simulink model "trajectory_tracking_simulation_on_kinematic_model_R2019b"  (R2019b)
settings: Solver=VariableStepAuto  StartTime=0.0  StopTime=20  RelTol=1e-3
InitFcn:
  | parameters_for_trajectory_tracking_simulation
StopFcn:
  | plot_trajectory_at_simulation_stop(out,true,0.5*half_wheel_base_for_model,false)
model workspace (MAT data in the model file):
  Current_Seg = Simulink.Signal
  Current_Seg.DataType = 'uint8'
  Current_Seg.Dimensions = -1
  Current_Seg.DimensionsMode = 'auto'
  Current_Seg.Complexity = 'auto'
  Current_Seg.SampleTime = -1
  Current_Seg.SamplingMode = 'auto'
  Current_Seg.InitialValue = '1'
  Current_Segment = Simulink.Signal
  Current_Segment.DataType = 'uint8'
  Current_Segment.Dimensions = -1
  Current_Segment.DimensionsMode = 'Fixed'
  Current_Segment.Complexity = 'real'
  Current_Segment.SampleTime = -1
  Current_Segment.SamplingMode = 'auto'
  Current_Segment.InitialValue = '0'
  Locked_Pos = Simulink.Signal
  Locked_Pos.DataType = 'uint8'
  Locked_Pos.Dimensions = -1
  Locked_Pos.DimensionsMode = 'auto'
  Locked_Pos.Complexity = 'auto'
  Locked_Pos.SampleTime = -1
  Locked_Pos.SamplingMode = 'auto'
  Locked_Pos.InitialValue = '0'
values from neighbouring files (symbols this model uses):
  half_wheel_base_for_controller = 0.125    [parameters_for_trajectory_tracking_simulation.m]
  half_wheel_base_for_model = 0.125    [parameters_for_trajectory_tracking_simulation.m]
  odometry_phi_initial = phi_initial    (= 0)    [parameters_for_trajectory_tracking_simulation.m]
  odometry_pose_covariance_initial = zeros(3,3)    [parameters_for_trajectory_tracking_simulation.m]
  odometry_theta_l_variance_scaling = (0.05)^2    (= 0.0025)    [parameters_for_trajectory_tracking_simulation.m]
  odometry_theta_r_variance_scaling = (0.05)^2    (= 0.0025)    [parameters_for_trajectory_tracking_simulation.m]
  odometry_x_p_initial = x_p_initial    (= 0.5)    [parameters_for_trajectory_tracking_simulation.m]
  odometry_y_p_initial = y_p_initial    (= 3)    [parameters_for_trajectory_tracking_simulation.m]
  phi_initial = 0 * (pi/180)    (= 0)    [development_of_path_planning.m]    (also in parameters_for_trajectory_tracking_simulation.m; path_planning_and_trajectory_generation.m = pose_initial(3))
  theta_l_initial = 0    [parameters_for_trajectory_tracking_simulation.m]
  theta_r_initial = 0    [parameters_for_trajectory_tracking_simulation.m]
  trajectory_description = [0.5, 3, 1, 3.5, pi/4 ... (first row only)    [path_planning_and_trajectory_generation.m]
  wheel_radius_left_for_controller = 0.050    (= 0.05)    [parameters_for_trajectory_tracking_simulation.m]
  wheel_radius_left_for_model = 0.050    (= 0.05)    [parameters_for_trajectory_tracking_simulation.m]
  wheel_radius_right_for_controller = 0.050    (= 0.05)    [parameters_for_trajectory_tracking_simulation.m]
  wheel_radius_right_for_model = 0.050    (= 0.05)    [parameters_for_trajectory_tracking_simulation.m]
  x_p_initial = 0.5    [development_of_path_planning.m]    (also in parameters_for_trajectory_tracking_simulation.m; path_planning_and_trajectory_generation.m = pose_initial(1))
  y_p_initial = 3.0    (= 3)    [development_of_path_planning.m]    (also in parameters_for_trajectory_tracking_simulation.m; path_planning_and_trajectory_generation.m = pose_initial(2))
settings Model: Creator=pbeuchat  LastModifiedBy=nicpa

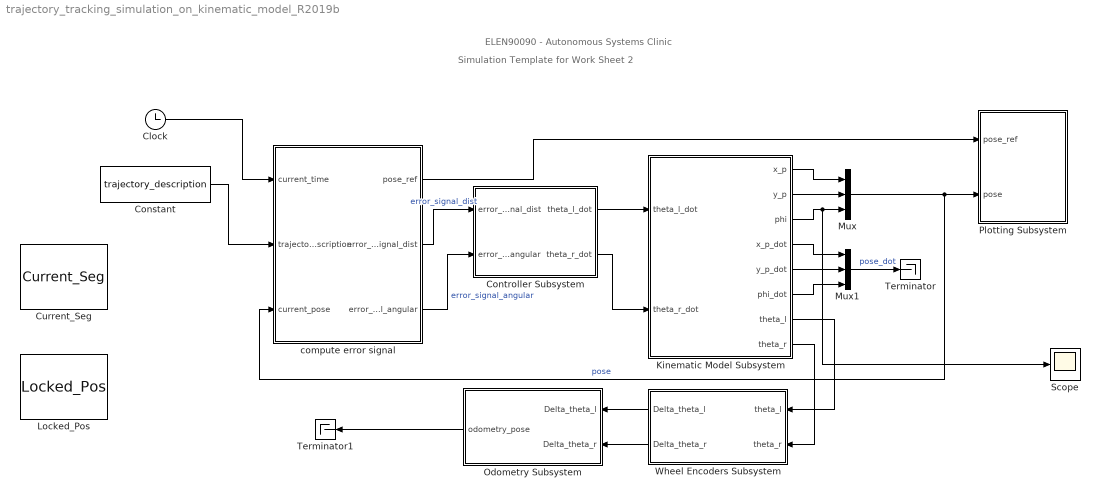
== system trajectory_tracking_simulation_on_kinematic_model_R2019b ==
  note: ELEN90090 - Autonomous Systems Clinic
  note: Simulation Template for Work Sheet 2
  Clock : Clock
  Constant : Constant  Value=trajectory_description
  Controller Subsystem : Subsystem
  Current_Seg : DataStoreMemory  DataStoreName=Current_Seg  ReadBeforeWriteMsg=warning  WriteAfterWriteMsg=warning  WriteAfterReadMsg=warning  InitialValue=1  ShowAdditionalParam=off  OutDataTypeStr=uint8  StateMustResolveToSignalObject=on
  Kinematic Model Subsystem : Subsystem
  Locked_Pos : DataStoreMemory  DataStoreName=Locked_Pos  ReadBeforeWriteMsg=warning  WriteAfterWriteMsg=warning  WriteAfterReadMsg=warning  ShowAdditionalParam=off  OutDataTypeStr=uint8  StateMustResolveToSignalObject=on
  Mux : Mux  Inputs=3
  Mux1 : Mux  Inputs=3
  Odometry Subsystem : Subsystem
  Plotting Subsystem : Subsystem
  Scope : Scope
  Terminator : Terminator
  Terminator1 : Terminator
  Wheel Encoders Subsystem : Subsystem
  compute error signal : MATLAB Function  TreatAsAtomicUnit=on
  wires:
  Kinematic Model Subsystem/1(x_p) -> Mux/1
  Kinematic Model Subsystem/2(y_p) -> Mux/2
  Mux/1 -> compute error signal/3(current_pose), Plotting Subsystem/2(pose)  "pose"
  Kinematic Model Subsystem/4(x_p_dot) -> Mux1/1
  Kinematic Model Subsystem/5(y_p_dot) -> Mux1/2
  Kinematic Model Subsystem/6(phi_dot) -> Mux1/3
  Mux1/1 -> Terminator/1  "pose_dot"
  compute error signal/2(error_signal_dist) -> Controller Subsystem/1("error_signal_dist ")  "error_signal_dist"
  Controller Subsystem/1(theta_l_dot) -> Kinematic Model Subsystem/1(theta_l_dot)
  Controller Subsystem/2(theta_r_dot) -> Kinematic Model Subsystem/2(theta_r_dot)
  compute error signal/1(pose_ref) -> Plotting Subsystem/1(pose_ref)
  Clock/1 -> compute error signal/1(current_time)
  Constant/1 -> compute error signal/2(trajectory_description)
  Kinematic Model Subsystem/7(theta_l) -> Wheel Encoders Subsystem/1(theta_l)
  Kinematic Model Subsystem/8(theta_r) -> Wheel Encoders Subsystem/2(theta_r)
  Wheel Encoders Subsystem/1(Delta_theta_l) -> Odometry Subsystem/1(Delta_theta_l)
  Wheel Encoders Subsystem/2(Delta_theta_r) -> Odometry Subsystem/2(Delta_theta_r)
  Odometry Subsystem/1(odometry_pose) -> Terminator1/1
  compute error signal/3(error_signal_angular) -> Controller Subsystem/2("error_signal_angular ")  "error_signal_angular"
  Kinematic Model Subsystem/3(phi) -> Scope/1, Mux/3

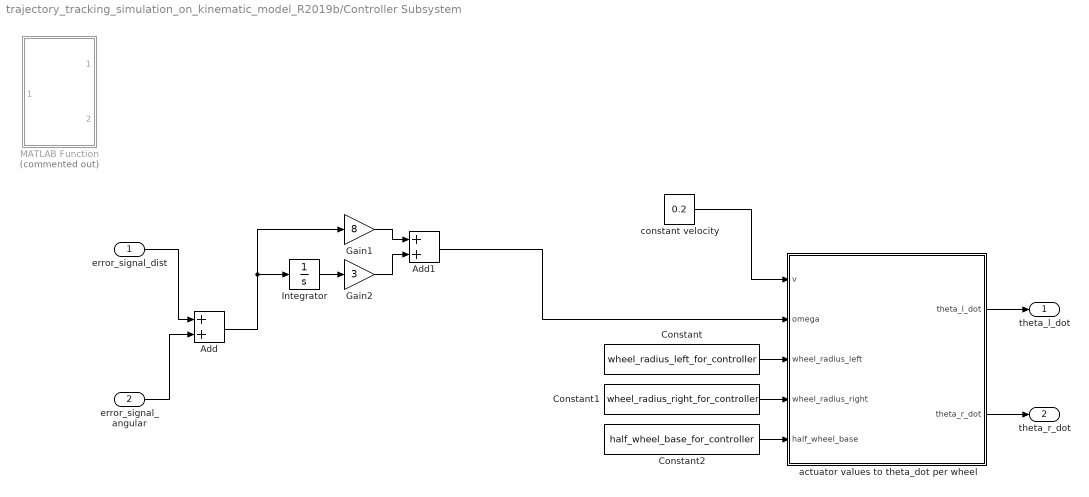
== system trajectory_tracking_simulation_on_kinematic_model_R2019b/Controller Subsystem ==
  "error_signal_dist " : Inport
  "error_signal_angular " : Inport  Port=2
  Add : Sum
  Add1 : Sum
  Constant : Constant  Value=wheel_radius_left_for_controller
  Constant1 : Constant  Value=wheel_radius_right_for_controller
  Constant2 : Constant  Value=half_wheel_base_for_controller
  Gain1 : Gain  Gain=8
  Gain2 : Gain  Gain=3
  Integrator : Integrator
  MATLAB Function : MATLAB Function  Commented=on  TreatAsAtomicUnit=on
  actuator values to theta_dot per wheel : MATLAB Function  TreatAsAtomicUnit=on
  "constant velocity " : Constant  Value=0.2  OutDataTypeStr=Inherit: Inherit via back propagation
  theta_l_dot : Outport
  theta_r_dot : Outport  Port=2
  wires:
  Constant/1 -> actuator values to theta_dot per wheel/3(wheel_radius_left)
  actuator values to theta_dot per wheel/2(theta_r_dot) -> theta_r_dot/1
  actuator values to theta_dot per wheel/1(theta_l_dot) -> theta_l_dot/1
  Constant2/1 -> actuator values to theta_dot per wheel/5(half_wheel_base)
  Constant1/1 -> actuator values to theta_dot per wheel/4(wheel_radius_right)
  "constant velocity "/1 -> actuator values to theta_dot per wheel/1(v)
  Add1/1 -> actuator values to theta_dot per wheel/2(omega)
  "error_signal_angular "/1 -> Add/2
  Integrator/1 -> Gain2/1
  Gain1/1 -> Add1/1
  Gain2/1 -> Add1/2
  "error_signal_dist "/1 -> Add/1
  Add/1 -> Gain1/1, Integrator/1

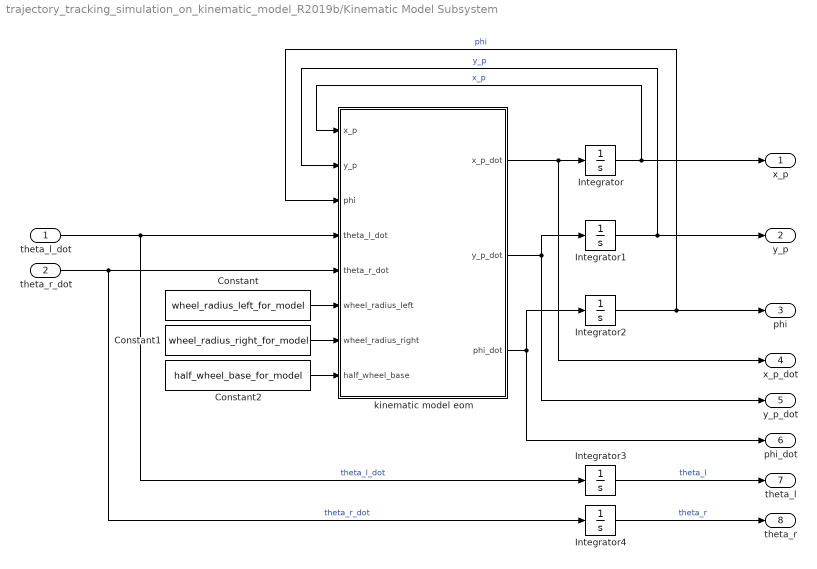
== system trajectory_tracking_simulation_on_kinematic_model_R2019b/Kinematic Model Subsystem ==
  theta_l_dot : Inport
  theta_r_dot : Inport  Port=2
  Constant : Constant  Value=wheel_radius_left_for_model
  Constant1 : Constant  Value=wheel_radius_right_for_model
  Constant2 : Constant  Value=half_wheel_base_for_model
  Integrator : Integrator  InitialCondition=x_p_initial
  Integrator1 : Integrator  InitialCondition=y_p_initial
  Integrator2 : Integrator  InitialCondition=phi_initial
  Integrator3 : Integrator  InitialCondition=theta_l_initial
  Integrator4 : Integrator  InitialCondition=theta_r_initial
  kinematic model eom : MATLAB Function  TreatAsAtomicUnit=on
  x_p : Outport
  y_p : Outport  Port=2
  phi : Outport  Port=3
  x_p_dot : Outport  Port=4
  y_p_dot : Outport  Port=5
  phi_dot : Outport  Port=6
  theta_l : Outport  Port=7
  theta_r : Outport  Port=8
  wires:
  theta_l_dot/1 -> kinematic model eom/4(theta_l_dot), Integrator3/1  "theta_l_dot"
  Integrator/1 -> kinematic model eom/1(x_p), x_p/1  "x_p"
  Constant1/1 -> kinematic model eom/7(wheel_radius_right)
  theta_r_dot/1 -> Integrator4/1, kinematic model eom/5(theta_r_dot)  "theta_r_dot"
  Constant/1 -> kinematic model eom/6(wheel_radius_left)
  kinematic model eom/1(x_p_dot) -> x_p_dot/1, Integrator/1
  kinematic model eom/2(y_p_dot) -> y_p_dot/1, Integrator1/1
  kinematic model eom/3(phi_dot) -> phi_dot/1, Integrator2/1
  Integrator1/1 -> y_p/1, kinematic model eom/2(y_p)  "y_p"
  Integrator2/1 -> phi/1, kinematic model eom/3(phi)  "phi"
  Constant2/1 -> kinematic model eom/8(half_wheel_base)
  Integrator4/1 -> theta_r/1  "theta_r"
  Integrator3/1 -> theta_l/1  "theta_l"

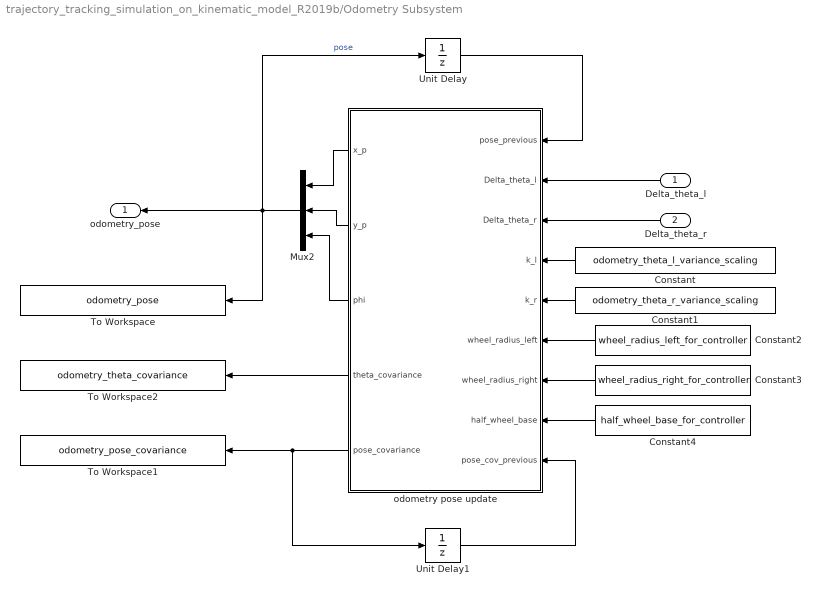
== system trajectory_tracking_simulation_on_kinematic_model_R2019b/Odometry Subsystem ==
  Delta_theta_l : Inport
  Delta_theta_r : Inport  Port=2
  Constant : Constant  Value=odometry_theta_l_variance_scaling
  Constant1 : Constant  Value=odometry_theta_r_variance_scaling
  Constant2 : Constant  Value=wheel_radius_left_for_controller
  Constant3 : Constant  Value=wheel_radius_right_for_controller
  Constant4 : Constant  Value=half_wheel_base_for_controller
  Mux2 : Mux  Inputs=3
  To Workspace : ToWorkspace  VariableName=odometry_pose  SaveFormat=Timeseries  SampleTime=-1
  To Workspace1 : ToWorkspace  VariableName=odometry_pose_covariance  SaveFormat=Timeseries  SampleTime=-1
  To Workspace2 : ToWorkspace  VariableName=odometry_theta_covariance  SaveFormat=Timeseries  SampleTime=-1
  Unit Delay : UnitDelay  InitialCondition=[odometry_x_p_initial;odometry_y_p_initial;odometry_phi_initial]  SampleTime=-1  HasFrameUpgradeWarning=on
  Unit Delay1 : UnitDelay  InitialCondition=odometry_pose_covariance_initial  SampleTime=-1  HasFrameUpgradeWarning=on
  odometry pose update : MATLAB Function  TreatAsAtomicUnit=on
  odometry_pose : Outport
  wires:
  Delta_theta_l/1 -> odometry pose update/2(Delta_theta_l)
  Delta_theta_r/1 -> odometry pose update/3(Delta_theta_r)
  odometry pose update/2(y_p) -> Mux2/2
  odometry pose update/1(x_p) -> Mux2/1
  Mux2/1 -> Unit Delay/1, odometry_pose/1, To Workspace/1  "pose"
  odometry pose update/3(phi) -> Mux2/3
  Unit Delay/1 -> odometry pose update/1(pose_previous)
  odometry pose update/5(pose_covariance) -> Unit Delay1/1, To Workspace1/1
  odometry pose update/4(theta_covariance) -> To Workspace2/1
  Constant/1 -> odometry pose update/4(k_l)
  Constant1/1 -> odometry pose update/5(k_r)
  Constant2/1 -> odometry pose update/6(wheel_radius_left)
  Constant3/1 -> odometry pose update/7(wheel_radius_right)
  Constant4/1 -> odometry pose update/8(half_wheel_base)
  Unit Delay1/1 -> odometry pose update/9(pose_cov_previous)

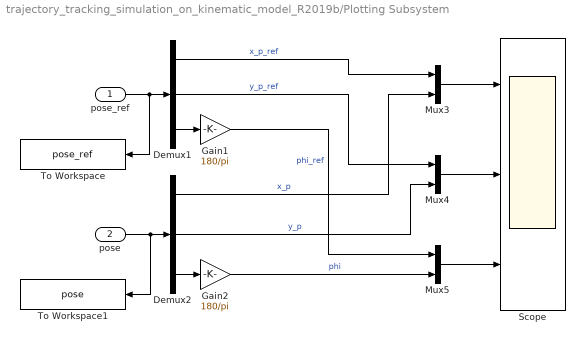
== system trajectory_tracking_simulation_on_kinematic_model_R2019b/Plotting Subsystem ==
  pose_ref : Inport
  pose : Inport  Port=2
  Demux1 : Demux  Outputs=3
  Demux2 : Demux  Outputs=3
  Gain1 : Gain  Gain=180/pi
  Gain2 : Gain  Gain=180/pi
  Mux3 : Mux  Inputs=2
  Mux4 : Mux  Inputs=2
  Mux5 : Mux  Inputs=2
  Scope : Scope  NumInputPorts=3
  To Workspace : ToWorkspace  VariableName=pose_ref  SaveFormat=Timeseries  SampleTime=-1
  To Workspace1 : ToWorkspace  VariableName=pose  SaveFormat=Timeseries  SampleTime=-1
  wires:
  Demux2/3 -> Gain2/1
  Mux3/1 -> Scope/1
  Gain2/1 -> Mux5/2  "phi"
  Demux1/3 -> Gain1/1
  Gain1/1 -> Mux5/1  "phi_ref"
  Mux5/1 -> Scope/3
  Demux2/2 -> Mux4/2  "y_p"
  pose/1 -> To Workspace1/1, Demux2/1
  Mux4/1 -> Scope/2
  Demux1/2 -> Mux4/1  "y_p_ref"
  Demux2/1 -> Mux3/2  "x_p"
  Demux1/1 -> Mux3/1  "x_p_ref"
  pose_ref/1 -> To Workspace/1, Demux1/1

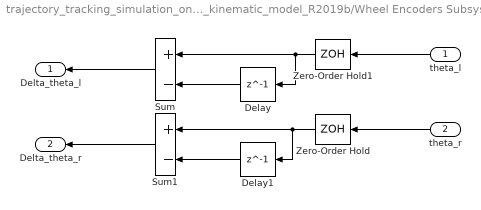
== system trajectory_tracking_simulation_on_kinematic_model_R2019b/Wheel Encoders Subsystem ==
  theta_l : Inport
  theta_r : Inport  Port=2
  Delay : Delay  DelayLength=1
  Delay1 : Delay  DelayLength=1
  Sum : Sum  Inputs=+-
  Sum1 : Sum  Inputs=+-
  Zero-Order Hold : ZeroOrderHold  SampleTime=0.01
  Zero-Order Hold1 : ZeroOrderHold  SampleTime=0.01
  Delta_theta_l : Outport
  Delta_theta_r : Outport  Port=2
  wires:
  theta_l/1 -> Zero-Order Hold1/1
  Sum1/1 -> Delta_theta_r/1
  theta_r/1 -> Zero-Order Hold/1
  Delay1/1 -> Sum1/2
  Zero-Order Hold/1 -> Sum1/1, Delay1/1
  Delay/1 -> Sum/2
  Sum/1 -> Delta_theta_l/1
  Zero-Order Hold1/1 -> Delay/1, Sum/1

== matlab function trajectory_tracking_simulation_on_kinematic_model_R2019b/Controller Subsystem/actuator values to theta_dot per wheel ==
  data: v input; theta_l_dot output; omega input; wheel_radius_left input; wheel_radius_right input; theta_r_dot output; half_wheel_base input
function [theta_l_dot , theta_r_dot] = ...
    actuators_to_theta_dot(...
        v ,...
        omega ,...
        wheel_radius_left ,...
        wheel_radius_right ,...
        half_wheel_base ...
    )
%  ---------------------------------------------------------------------  %
%% DESCRIPTION: THIS FUNCTION SHOULD CONVERT THE "v" AND "omega" ACTUATORS
%% TO DESIRED ANGULAR VELOCITY OF EACH WHEEL
%
%  INPUT ARGUMENTS:
%  v                    Forward velocity of the robot, in meters/second
%  omega                Angular velocity of the robot, in radians/second
%  wheel_radius_left    Radius of the left-hand wheel, in meters
%  wheel_radius_right   Radius of the right-hand wheel, in meters
%  half_wheel_base      Half the distance between the wheels, in meters
%
%  RETURN VARIABLES:
%  theta_l_dot    Angular velocity of the left-hand wheel, in radians/second
%  theta_r_dot    Angular velocity of the right-hand wheel, in radians/second
%
%  ---------------------------------------------------------------------  %

%% REPLACE THE CODE BELOW WITH THE CONVERSION
%simplified actuation

theta_l_dot = (v / wheel_radius_left) - (half_wheel_base * omega / wheel_radius_left);
%theta_l_dot = (v / wheel_radius_left);

theta_r_dot = (v / wheel_radius_right) + (half_wheel_base * omega / wheel_radius_right);

% %symbolic variables for equations solving 
% syms theta_l_dot_sym theta_r_dot_sym
% 
% %set up simultaneous equations
% eqn1 = (wheel_radius_left * theta_l_dot_sym / 2) + (wheel_radius_right * theta_r_dot_sym / 2) == v;
% eqn2 = (wheel_radius_right * theta_r_dot_sym / (2 * half_wheel_base)) - (wheel_radius_left * theta_l_dot_sym / (2 * half_wheel_base)) == omega;
% 
% %solve simultaneous equations 
% sol = solve([eqn1 eqn2], [theta_l_dot_sym theta_r_dot_sym]);
% 
% theta_l_dot = sol.theta_l_dot_sym;
% theta_r_dot = sol.theta_r_dot_sym;

== matlab function trajectory_tracking_simulation_on_kinematic_model_R2019b/Kinematic Model Subsystem/kinematic model eom ==
  data: x_p input; x_p_dot output; y_p input; phi input; theta_l_dot input; theta_r_dot input; y_p_dot output; phi_dot output; wheel_radius_left input; wheel_radius_right input; half_wheel_base input
function [x_p_dot,y_p_dot,phi_dot] = ...
    kinematic_model_eom(...
        x_p ,...
        y_p ,...
        phi ,...
        theta_l_dot ,...
        theta_r_dot ,...
        wheel_radius_left ,...
        wheel_radius_right ,...
        half_wheel_base ...
    )
%  ---------------------------------------------------------------------  %
%% DESCRIPTION: THIS FUNCTION SHOULD IMPLEMENT THE EQUATIONS OF MOTION
%% FOR THE KINEMATIC MODEL
%
%  INPUT ARGUMENTS:
%  x_p                  Intertial frame x-coordinate of the robot
%  y_p                  Intertial frame y-coordinate of the robot
%  phi                  Heading angle of the robot, in radians
%  theta_l_dot          Angular velocity of the left-hand wheel, in radians/second
%  theta_r_dot          Angular velocity of the right-hand wheel, in radians/second
%  wheel_radius_left    Radius of the left-hand wheel, in meters
%  wheel_radius_right   Radius of the right-hand wheel, in meters
%  half_wheel_base      Half the distance between the wheels, in meters
%
%  RETURN VARIABLES:
%  x_p_dot    Intertial frame x-coordinate velocity of the robot
%  y_p_dot    Intertial frame y-coordinate velocity of the robot
%  phi_dot    Heading anglular velocity of the robot
%
%  ---------------------------------------------------------------------  %

%% REAPLCE THE CODE BELOW WITH THE KINEMATIC MODEL
%transform from body frame to inertial frame
R_body_inertial = [cos(phi) -sin(phi) 0; sin(phi) cos(phi) 0; 0 0 1];

%note: assuming wheel_radius_left and wheel_radius right are the same. ALSO
%IF THEY ARENT THE SAME THIS MAY NOT BE THE CORRECT WAY TO PUT IT IN
wheel_params_matrix = [wheel_radius_left/2 wheel_radius_right/2; 0 0; 
    -wheel_radius_left/(2*half_wheel_base) wheel_radius_right/(2*half_wheel_base)];

wheel_velocities = [theta_l_dot; theta_r_dot];

velocities = R_body_inertial * wheel_params_matrix * wheel_velocities;


x_p_dot = velocities(1);
y_p_dot = velocities(2);
phi_dot = velocities(3);

== matlab function trajectory_tracking_simulation_on_kinematic_model_R2019b/compute error signal ==
  settings: updateMethod=DISCRETE
  data: pose_ref output; current_time input; trajectory_description input; error_signal_dist output; current_pose input; Current_Seg data_store_memory; Locked_Pos data_store_memory; error_signal_angular output
function [pose_ref , error_signal_dist, error_signal_angular] = ...
    compute_error_signal(...
        current_time ,...
        trajectory_description, ...
        current_pose)...
%  ---------------------------------------------------------------------  %
%% DESCRIPTION: THIS FUNCTION SHOULD GENERATE AN ERROR SIGNAL FOR X, Y AND THE HEADING
%
%  INPUT ARGUMENTS:
%  current_time    The current simulation time, in seconds
%
%  trajectory_description
%                  This is a matrix that specifies the interconnection of
%                  straight line segments that define the trajectory to
%                  follow as a function of time. Each row corresponds to a
%                  line segment, describing the start and end point of 
%                  the segment and the target heading i.e. each row is:
%                  [start_x start_y end_x end_y heading]
%
%  current_pose    A column vector of length 3 with the current pose of the
%                  robot, i.e.:
%                  current_pose(1) = x_p measurement, in meters
%                  current_pose(2) = y_p measurement, in meters
%                  current_pose(3) = heading angle measurement, in radians
%
% RETURN VARIABLE:
% pose_ref        A column vecotr of length 3 with the current reference
%                 along the trajectory, i.e.:
%                 pose_ref(1) = reference for x_p, in meters
%                 pose_ref(2) = reference for y_p, in meters
%                 pose_ref(3) = reference for heading angle, in radians
%
% error_signal    A column vector that is passed to the controller
%                 sub-system. You can give this vector any length you
%                 choose, but remember to ensure that the controller
%                 sub-system is compatible with the error signal "y" that
%                 you return.
%                 It is good practice to define here in the comments what
%                 the components of the vector "y" respresent:
%                 y(1) = shortest distance from robot to line
%                 y(2) = angular error between robot and line
%NOTE: splitting it up into two components because passing it as a vector
%was causing errors
%  ---------------------------------------------------------------------  %



%  ---------------------------------------------------------------------  %
%% INITIALISE THE SIZE OF "y"

% This is not strictly necessary, but it is good practice to assist with
% debugging.

%error_signal = zeros(2,1);

pose_ref = zeros(3,1);


%  ---------------------------------------------------------------------  %
%% EXTRACT THE COMPONENTS OF "current_pose_measurement"

current_x_p  = current_pose(1);
current_y_p  = current_pose(2);
current_phi  = current_pose(3);


%  ---------------------------------------------------------------------  %
%% REPLACE THE CODE BELOW WITH THE YOUR ALGORITHM FOR COMPUTING THE
%% ERROR SIGNAL FROM THE TRAJECTORY DESCRIPTION

%trajectory_description rows: [start_x start_y end_x end_y heading]

%follow each line segment until you are within a distance of EPSILON from 
%the end of the line segment, at which point stop and rotate until within
%a certain angular displacement from the heading of the new line segment,
%then follow that new line segment

%track a global variable for the current segment and increment it when you
%reach the end of a segment, initial value is 1
global Current_Seg;

%global variable for whether the robot's position is locked in place
global Locked_Pos;

%constants to define how close you should be to the end of a segment before
%going to the next one
EPSILON = 0.05; %metres, change this
ANGULAR_EPSILON = 0.05; %rad, change this

%get the number of line segments (the rows in trajectory_description)
[num_segments, cols] = size(trajectory_description);

%generate the target x,y and heading based on the current segment
%Current_Seg
pose_ref(1) = trajectory_description(Current_Seg, 3); %x ref
pose_ref(2) = trajectory_description(Current_Seg, 4); %y ref
% pose_ref(3) = trajectory_description(Current_Seg, 5); %phi ref
pose_ref(3) = atan2(pose_ref(2) - trajectory_description(Current_Seg, 2), pose_ref(1) - trajectory_description(Current_Seg, 1)); %phi ref

%compute euclidean distance to the end of the current line segment
dist_to_end_of_seg = sqrt( ((current_x_p - pose_ref(1))^2) + ((current_y_p - pose_ref(2))^2));

%go to the next path segment if you are close enough to the end of the
%current segment. make sure when this happens, you lock the x and y 
%references to where they are until you've turned to face the new path
if ((dist_to_end_of_seg < EPSILON) && (Current_Seg <= num_segments)) 
    Current_Seg = Current_Seg + 1;
    Locked_Pos = uint8(1);    
end

%unlock the position if you are facing down the new path
if (abs((current_phi - pose_ref(3))) < ANGULAR_EPSILON)
    Locked_Pos = uint8(0);
end

%calculate perpendicular distance to track. NOTE: denote the start of the
%line segment as point A, the end as B, the location of the robot as C
%and the closest point on the line from the robot as D

%find vector from start of line segment to current position
Vac1 = current_pose(1) - trajectory_description(Current_Seg,1);
Vac2 = current_pose(2) - trajectory_description(Current_Seg,2);
Vac = [Vac1 Vac2];

%find vector from start to end of line segment
Vab1 = trajectory_description(Current_Seg,3) - trajectory_description(Current_Seg,1);
Vab2 = trajectory_description(Current_Seg,4) - trajectory_description(Current_Seg,2);
Vab = [Vab1 Vab2];

%find vector from start of line segment to the closest point on the line
%from the current position
Vad = (dot(Vac,Vab) / (norm(Vab)^2)) .* Vab; %is this the right way to get Vad ? send help

%now get Vdc (the vector from the closest point on the line to the robot)
Vdc = -Vad + Vac;

%% Work out direction of robot from the line
%augment Vab and Vdc with a z axis component of 0
temp_Vab_x = Vab(1);
temp_Vab_y = Vab(2);
Vab = [temp_Vab_x temp_Vab_y 0].';

temp_Vdc_x = Vdc(1);
temp_Vdc_y = Vdc(2);
Vdc = [temp_Vdc_x temp_Vdc_y 0].';

%take the cross product of the segment direction vector (Vab) with Vdc
%(vector from the line to the robot).
%the z-coordinate sign gives the direction of the control action
direction_indicator = cross(Vab, Vdc);
direction = -sign(direction_indicator(3));

%the magnitude of Vdc is the shortest distance to the line 
short_dist = norm(Vdc);

%% return the error signals
%perpendicular distance of the robot from the line 
error_signal_dist = direction * short_dist; %error_signal(1)
%how misaligned the robot is to the line segment. reset to 0 when it is
%greater than 2*pi or less than -2*pi
error_signal_angular = rem(pose_ref(3), 2*pi) - rem(current_phi, 2*pi); %error_signal_angular

end

== matlab function trajectory_tracking_simulation_on_kinematic_model_R2019b/Odometry Subsystem/odometry pose update ==
  data: pose_previous input; x_p output; Delta_theta_l input; Delta_theta_r input; y_p output; phi output; theta_covariance output; pose_covariance output; k_l input; k_r input; wheel_radius_left input; wheel_radius_right input; half_wheel_base input; pose_cov_previous input

% function [output] =
%                    input 

function [ x_p , y_p , phi , theta_covariance , pose_covariance ] = ...
    odometry_pose_update(...
        pose_previous ,...
        Delta_theta_l ,...
        Delta_theta_r ,...
        k_l ,...
        k_r ,...
        wheel_radius_left ,...
        wheel_radius_right ,...
        half_wheel_base ,...
        pose_cov_previous ...
    )
%  ---------------------------------------------------------------------  %
%% DESCRIPTION: THIS FUNCTION SHOULD CONVERT THE "v" AND "omega" ACTUATORS
%% TO DESIRED ANGULAR VELOCITY OF EACH WHEEL
%
%  INPUT ARGUMENTS:
%  pose_previous        Previous pose output of this function
%  Delta_theta_l        Change in left-hand wheel position, in radians
%  Delta_theta_r        Change in right-hand wheel position, in radians
%  k_l                  Constant of proportionality for left-hand wheel errors
%  k_r                  Constant of proportionality for right-hand wheel errors
%  wheel_radius_left    Radius of the left-hand wheel, in meters
%  wheel_radius_right   Radius of the right-hand wheel, in meters
%  half_wheel_base      Half the distance between the wheels, in meters
%  pose_cov_previous    Previous pose covariance output of this function
%
%  RETURN VARIABLES:
%  x_p                 Odometry estimate of tntertial frame x-coordinate
%  y_p                 Odometry estimate of tntertial frame y-coordinate
%  phi                 Heading angle of the robot, in radians
%  theta_covariance    Covariance matrix (2x2) of the encoder measurements
%  pose_covariance     Covariance matrix (3x3) of the pose estimate
%
%  ---------------------------------------------------------------------  %

%  ---------------------------------------------------------------------  %

%% INITIALISE THE SIZE OF "y"

% This is not strictly necessary, but it is good practice to assist with
% debugging.

% Initialise the output variables:
x_p = 0;
y_p = 0;
phi = 0;
pose_covariance = zeros(3,3);
theta_covariance = zeros(2,2);


%  ---------------------------------------------------------------------  %
%% EXTRACT THE COMPONENTS OF "current_pose_measurement"

% Extract the location and heading angle of the previous pose
x_p_previous = pose_previous(1);
y_p_previous = pose_previous(2);
phi_previous = pose_previous(3);


%  ---------------------------------------------------------------------  %
%% REPLACE THE CODE BELOW WITH THE ODOMETRY COMPUTATIONS

% Put the pose update into the return variables
% x_p(1) = 0;
% y_p(1) = 0;
% phi(1) = 0;


delta_s = (wheel_radius_left * Delta_theta_l + wheel_radius_right * Delta_theta_r) / 2;
delta_phi = (wheel_radius_right * Delta_theta_r - wheel_radius_left * Delta_theta_l) / (2*half_wheel_base);

x_p(1) = x_p_previous + delta_s * cos(phi_previous + 0.5 * delta_phi);
y_p(1) = y_p_previous + delta_s * sin(phi_previous + 0.5 * delta_phi);
phi(1) = phi_previous + delta_phi;

% Put the covariance of the wheel measurements into the return variable
theta_covariance(1,1) = k_l * abs(Delta_theta_l);
theta_covariance(2,2) = k_r * abs(Delta_theta_r);


% Put the covariance of the pose into the return variable
Jacobian_p = eye(3);
Jacobian_theta_first_column = [wheel_radius_left/2 * cos(phi_previous + 0.5 * delta_phi) + (wheel_radius_left * Delta_theta_l)/2 * (-1) * sin(phi_previous + 0.5 * delta_phi)*(-wheel_radius_left/(4*half_wheel_base));
                                wheel_radius_left/2 * sin(phi_previous + 0.5 * delta_phi)+ (wheel_radius_left * Delta_theta_l)/2 * cos(phi_previous + 0.5 * delta_phi)*(-wheel_radius_left/(4*half_wheel_base));
                                -wheel_radius_left/(2*half_wheel_base)];
                            
Jacobian_theta_second_column = [wheel_radius_right/2 * cos(phi_previous + 0.5 * delta_phi) + (wheel_radius_right * Delta_theta_r)/2 * (-1) * sin(phi_previous + 0.5 * delta_phi)*(wheel_radius_right/(4*half_wheel_base));
                                wheel_radius_right/2 * sin(phi_previous + 0.5 * delta_phi)+ (wheel_radius_right * Delta_theta_r)/2 * cos(phi_previous + 0.5 * delta_phi)*(wheel_radius_right/(4*half_wheel_base));
                                wheel_radius_right/(2*half_wheel_base)];  
                            
Jacobian_theta = [Jacobian_theta_first_column Jacobian_theta_second_column]; 

pose_covariance(1:3,1:3) = Jacobian_p * pose_cov_previous * transpose(Jacobian_p) + Jacobian_theta * theta_covariance * transpose(Jacobian_theta);

== matlab function trajectory_tracking_simulation_on_kinematic_model_R2019b/Controller Subsystem/MATLAB Function ==
  data: error_signal input; perp_dist output; angle_error output
function [perp_dist, angle_error] = fcn(error_signal)

perp_dist = error_signal(1);
angle_error = error_signal(2);
end
